simulink model "CSE1_DP"  (R2014a)
settings: Solver=ode4  StartTime=0.0  StopTime=time  FixedStep=h  RelTol=1e-3
values from neighbouring files (symbols this model uses):
  head_pitch = 0    [run_file.m]
  Head_roll = 0    [run_file.m]
  head_yaw = 0    [run_file.m]
  K_2_psi = 30    [run_file.m]
  K_2_x = 30    [run_file.m]
  K_2_y = 30    [run_file.m]
  K_3_psi = 2    [run_file.m]
  K_3_x = 2    [run_file.m]
  K_3_y = 2    [run_file.m]
  K_4_psi = 2    [run_file.m]
  K_4_x = 2    [run_file.m]
  K_4_y = 2    [run_file.m]
  K_d_psi = 8    [run_file.m]
  K_d_x = 8    [run_file.m]
  K_d_y = 8    [run_file.m]
  K_ff_r = 0    [run_file.m]
  K_ff_r_dot = 0    [run_file.m]
  K_ff_u = 0    [run_file.m]
  K_ff_u_dot = 0    [run_file.m]
  K_ff_v = 0    [run_file.m]
  K_ff_v_dot = 0    [run_file.m]
  K_i_psi = 0    [run_file.m]
  K_i_x = 0    [run_file.m]
  K_i_y = 0    [run_file.m]
  K_p_psi = 3    [run_file.m]
  K_p_x = 3    [run_file.m]
  K_p_y = 3    [run_file.m]
  K_r = 0.5    [run_file.m]
  K_u = 1    [run_file.m]
  K_v = 0.5    [run_file.m]
  L = 1    [plot_script.m]    (also in run_file.m = diag([1 1 1]))
  M = [m_11 0    0 ... (first row only)    [run_file.m]
  psi_0 = 1    [run_file.m]
  psi_ref = ref(4,:)    [plot_script.m]    (also in run_file.m = 3.14159265359)
  v_max = [0.3 0.1 1]    [run_file.m]
  w_d_psi = 2    [run_file.m]
  w_d_psi_2 = 2    [run_file.m]
  w_d_x = 1    [run_file.m]
  w_d_x_2 = 1    [run_file.m]
  w_d_y = 1    [run_file.m]
  w_d_y_2 = 1    [run_file.m]
  x_0 = 5    [run_file.m]
  x_ref = ref(2,:)    [plot_script.m]    (also in run_file.m = 4)
  y_0 = 5    [run_file.m]
  y_ref = ref(3,:)    [plot_script.m]    (also in run_file.m = 3)
  zeta_psi = 1    [run_file.m]
  zeta_psi_2 = 1    [run_file.m]
  zeta_x = 1    [run_file.m]
  zeta_x_2 = 1    [run_file.m]
  zeta_y = 1    [run_file.m]
  zeta_y_2 = 1    [run_file.m]
libraries: marine_gnc x15, simulink x2
(part 2 of 2)

== matlab function CSE1_DP/Input/Guidance gains/Postirion guidance/diag ==
  data: w_d output; w_d_vector input
function w_d = fcn(w_d_vector)
%#codegen

w_d = diag(w_d_vector);

== matlab function CSE1_DP/Input/Guidance gains/Postirion guidance/diag1 ==
  data: Zeta output; zeta_vector input
function Zeta = fcn(zeta_vector)
%#codegen

Zeta = diag(zeta_vector);

== matlab function CSE1_DP/Input/Observer Gains/MATLAB Function2 ==
  data: K_d output; K_d1 input
function K_d = fcn(K_d1)
%#codegen

K_d = diag(K_d1);

== matlab function CSE1_DP/Input/Control Gains/MATLAB Function3 ==
  data: K_p output; K_p1 input
function K_p = fcn(K_p1)
%#codegen

K_p = diag(K_p1);

== matlab function CSE1_DP/Input/Control Gains/MATLAB Function4 ==
  data: K_p output; K_p1 input
function K_p = fcn(K_p1)
%#codegen

K_p = diag(K_p1);

== matlab function CSE1_DP/Navigation /Derivative filter/MATLAB Function ==
  data: a input; eta_filtered output; eta input; eta_filtered_prev input
function eta_filtered = fcn(a,eta,eta_filtered_prev)

eta_filtered = a*eta + (1-a)*eta_filtered_prev;

== matlab function CSE1_DP/Navigation /Derivative filter/MATLAB Function1 ==
  data: h input; eta_dot output; eta input; eta_prev input
function eta_dot  = fcn(h,eta,eta_prev)

eta_dot = (eta-eta_prev)./h;

== matlab function CSE1_DP/Navigation /Derivative filter/MATLAB Function2 ==
  data: a input; eta_dot_filtered output; eta_dot input; eta_dot_filtered_prev input
function eta_dot_filtered = fcn(a,eta_dot,eta_dot_filtered_prev)

eta_dot_filtered = a*eta_dot + (1-a)*eta_dot_filtered_prev;

== matlab function CSE1_DP/Navigation /Derivative filter/MATLAB Function3 ==
  data: eta_dot input; nu output; psi input
function nu = fcn(eta_dot,psi)

R_inv = [cos(psi)  sin(psi) 0
         -sin(psi) cos(psi) 0
         0         0        1];
nu = R_inv*eta_dot;

== matlab function CSE1_DP/Guidance/Vel Reference model1/w_d*w_d ==
  data: w_d input; y output
function y = fcn(w_d)
%#codegen

y = w_d*w_d;

== matlab function CSE1_DP/Guidance/Vel Reference model1/w_d*w_d1 ==
  data: w_d input; y output; zeta input
function y = fcn(w_d,zeta)
%#codegen

y = 2*zeta*w_d;

== matlab function CSE1_DP/Guidance/Vel Reference model1/w_d^-2 ==
  data: w_d input; y output
function y = fcn(w_d)
%#codegen

y = w_d^-2;

== matlab function CSE1_DP/Guidance/Vel Reference model1/w_d^3 ==
  data: w_d input; y output
function y = fcn(w_d)
%#codegen

y = w_d^3;

== matlab function CSE1_DP/Input/Guidance gains/Velocity guidance/diag ==
  data: w_d output; w_d_vector input
function w_d = fcn(w_d_vector)
%#codegen

w_d = diag(w_d_vector);

== matlab function CSE1_DP/Input/Guidance gains/Velocity guidance/diag1 ==
  data: Zeta output; zeta_vector input
function Zeta = fcn(zeta_vector)
%#codegen

Zeta = diag(zeta_vector);

== matlab function CSE1_DP/Input/Gesture based ctrl/MATLAB Function4 ==
  data: K_p output; K_p1 input
function K_p = fcn(K_p1)
%#codegen

K_p = diag(K_p1);
